simulink model "OneCircuit_3a"  (R2017b)
settings: Solver=VariableStepAuto  StartTime=0.0  StopTime=864000000  RelTol=1e-3
libraries: instrumentlib x2, svdutilitieslib x1
settings Model: Creator=Bruger  LastModifiedBy=koch

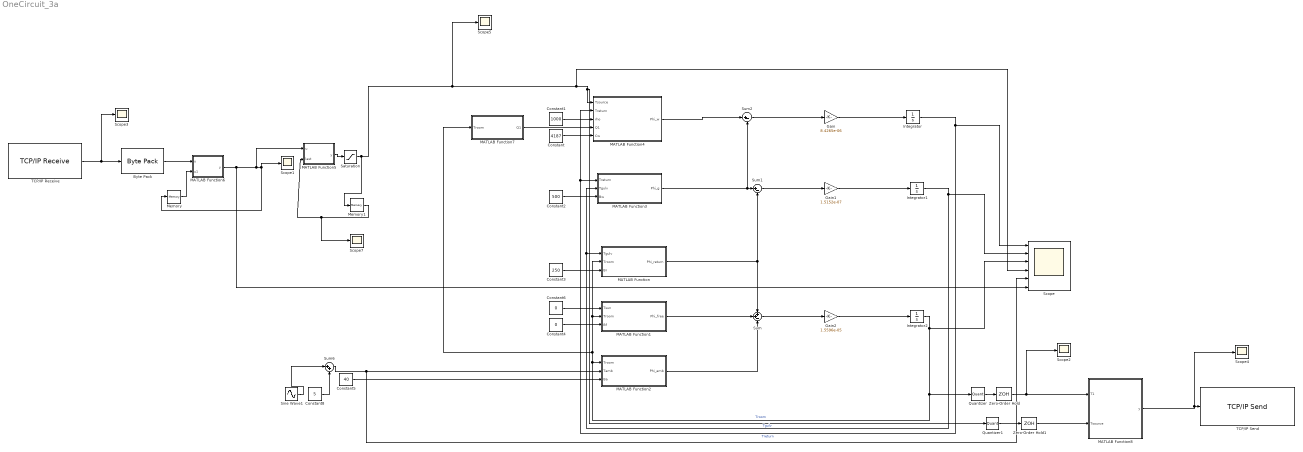
== system OneCircuit_3a ==
  Byte Pack : svdutilitieslib/Byte Pack  datatypes={'uint8'}  byteAlign=1  blockPlatform=arduinoert
      settings: SourceProductName=Simulink Support Package for Arduino Hardware  SourceProductBaseCode=ARDUINO
  Constant : Constant  Value=4187
  Constant1 : Constant  Value=1000
  Constant2 : Constant  Value=500
  Constant3 : Constant  Value=250
  Constant4 : Constant  Value=0
  Constant5 : Constant  Value=40
  Constant6 : Constant  Value=0
  Constant8 : Constant  Value=5
  Gain : Gain  Gain=8.4265e-06
  Gain1 : Gain  Gain=1.5152e-07
  Gain2 : Gain  Gain=1.5596e-05
  Integrator : Integrator  InitialCondition=16
  Integrator1 : Integrator  InitialCondition=16
  Integrator2 : Integrator  InitialCondition=16
  MATLAB Function : MATLAB Function  TreatAsAtomicUnit=on
  MATLAB Function1 : MATLAB Function  TreatAsAtomicUnit=on
  MATLAB Function2 : MATLAB Function  TreatAsAtomicUnit=on
  MATLAB Function3 : MATLAB Function  TreatAsAtomicUnit=on
  MATLAB Function4 : MATLAB Function  TreatAsAtomicUnit=on
  MATLAB Function5 : MATLAB Function  TreatAsAtomicUnit=on
  MATLAB Function6 : MATLAB Function  TreatAsAtomicUnit=on
  MATLAB Function7 : MATLAB Function  TreatAsAtomicUnit=on
  MATLAB Function8 : MATLAB Function  TreatAsAtomicUnit=on
  Memory : Memory
  Memory1 : Memory  InitialCondition=35  InheritSampleTime=on
  Quantizer : Quantizer  QuantizationInterval=0.1
  Quantizer1 : Quantizer  QuantizationInterval=0.1
  Saturation : Saturate  UpperLimit=45  LowerLimit=20
  Scope : Scope  NumInputPorts=6
  Scope{1..5,7} (6 alike) : Scope
  Sine Wave1 : Sin  Amplitude=3  Frequency=0.000004272205  SampleTime=0
  Sum : Sum  Inputs=++-
  Sum1 : Sum  Inputs=|+-
  Sum2 : Sum  Inputs=|+-
  Sum6 : Sum  Inputs=|++
  TCP/IP Receive : instrumentlib/TCP//IP Receive  Host=localhost  Port=50000  DataSize=[1 1]  EnableBlockingMode=on  Timeout=10  SampleTime=600  DataType=uint8  ByteOrder=BigEndian
      settings: SourceProductName=Instrument Control Toolbox
  TCP/IP Send : instrumentlib/TCP//IP Send  Host=localhost  Port=50001  EnableBlockingMode=on  Timeout=10  ByteOrder=LittleEndian
      settings: SourceProductName=Instrument Control Toolbox
  Zero-Order Hold : ZeroOrderHold  SampleTime=-1
  Zero-Order Hold1 : ZeroOrderHold  SampleTime=-1
  wires:
  Sine Wave1/1 -> Sum6/1
  Constant8/1 -> Sum6/2
  Integrator2/1 -> Scope/3, Quantizer/1, MATLAB Function2/1(Troom), MATLAB Function7/1(Troom), MATLAB Function/2(Troom), MATLAB Function1/2(Troom)  "Troom"
  MATLAB Function2/1(Phi_amb) -> Sum/3
  Constant4/1 -> MATLAB Function1/3(Bf)
  Sum2/1 -> Gain/1
  MATLAB Function1/1(Phi_free) -> Sum/2
  Integrator1/1 -> Scope/2, MATLAB Function/1(Tgulv), MATLAB Function3/2(Tgulv)  "Tgulv"
  MATLAB Function4/1(Phi_w) -> Sum2/1
  Constant2/1 -> MATLAB Function3/3(Bw)
  MATLAB Function3/1(Phi_g) -> Sum2/2, Sum1/1
  MATLAB Function/1(Phi_return) -> Sum/1, Sum1/2
  MATLAB Function7/1(Q1) -> MATLAB Function4/4(Q1)
  Constant1/1 -> MATLAB Function4/3(rho)
  Gain2/1 -> Integrator2/1
  Gain1/1 -> Integrator1/1
  Constant6/1 -> MATLAB Function1/1(Tsun)
  Constant/1 -> MATLAB Function4/5(Cw)
  Sum/1 -> Gain2/1
  Integrator/1 -> Scope/1, MATLAB Function4/2(Treturn), MATLAB Function3/1(Treturn)  "Treturn"
  Gain/1 -> Integrator/1
  Constant5/1 -> MATLAB Function2/3(Ba)
  Constant3/1 -> MATLAB Function/3(Br)
  Sum1/1 -> Gain1/1
  Sum6/1 -> Scope/5, MATLAB Function2/2(Tamb)
  MATLAB Function6/1(y) -> Scope/6, MATLAB Function5/1(u), Memory/1, Scope1/1
  TCP/IP Receive/1 -> Scope3/1, Byte Pack/1
  Memory/1 -> MATLAB Function6/2(u1)
  Byte Pack/1 -> MATLAB Function6/1(u)
  Quantizer/1 -> Zero-Order Hold/1
  Zero-Order Hold/1 -> Scope2/1, MATLAB Function8/1(T1)
  MATLAB Function8/1(y) -> Scope4/1, TCP/IP Send/1
  MATLAB Function5/1(y) -> Saturation/1
  Memory1/1 -> Scope7/1, MATLAB Function5/2(last)
  Saturation/1 -> Memory1/1, Scope5/1, Scope/4, Quantizer1/1, MATLAB Function4/1(Tsource)
  Quantizer1/1 -> Zero-Order Hold1/1
  Zero-Order Hold1/1 -> MATLAB Function8/2(Tsource)

== matlab function OneCircuit_3a/MATLAB Function1 ==
  data: Tsun input; Phi_free output; Troom input; Bf input
function Phi_free = fcn(Tsun,Troom,Bf)

Phi_free = Bf * ( Tsun-Troom)

== matlab function OneCircuit_3a/MATLAB Function ==
  data: Tgulv input; Phi_return output; Troom input; Br input
function Phi_return = fcn(Tgulv,Troom,Br)

Phi_return = Br * ( Tgulv-Troom)

== matlab function OneCircuit_3a/MATLAB Function2 ==
  data: Troom input; Tamb input; Phi_amb output; Ba input
function Phi_amb = fcn(Troom,Tamb,Ba)

Phi_amb = Ba * ( Troom-Tamb)

== matlab function OneCircuit_3a/MATLAB Function3 ==
  data: Treturn input; Tgulv input; Phi_g output; Bw input
function Phi_g= fcn(Treturn,Tgulv,Bw)

Phi_g = Bw * ( Treturn-Tgulv)

== matlab function OneCircuit_3a/MATLAB Function4 ==
  data: Tsource input; Treturn input; Phi_w output; rho input; Q1 input; Cw input
function Phi_w= fcn(Tsource,Treturn,rho,Q1,Cw)

Phi_w = rho*Q1 *Cw* ( Tsource-Treturn)

== matlab function OneCircuit_3a/MATLAB Function5 ==
  data: u input; y output; last input
function y = fcn(u,last)

if u < 2
y = last
elseif 1 < u && u < 3 
    y=last -0.005
elseif 2 < u 
    y = last+0.005
else
    y=last
end

== matlab function OneCircuit_3a/MATLAB Function6 ==
  data: u input; y output; u1 input
function y = fcn(u,u1)

u = double(u);

if u > 0
    y = u;
else
    y = u1;
end

== matlab function OneCircuit_3a/MATLAB Function7 ==
  data: Troom input; Q1 output
function Q1 = fcn(Troom)

if Troom < 20
    Q1 = 0.000027777778
else 
    Q1 = 0.000027777778 
end

== matlab function OneCircuit_3a/MATLAB Function8 ==
  data: T1 input; y output; Tsource input
function y = fcn(T1, Tsource)


y = [T1, 4.5, 4.6, 4.7, Tsource];
